simulink model "Long_Transmission_Line_Model"  (R2024b)
settings: Solver=VariableStepAuto  StartTime=0.0  StopTime=0.1  RelTol=1e-3
libraries: spsRMSLib x4, spsPower3phInstantaneousLib x2, spsThreePhaseVIMeasurementLib x2, spsDistributedParametersLineLib x1, spsThreePhaseSeriesRLCLoadLib x1, spsThreePhaseSourceLib x1, sps_lib x1
settings Model: Creator=vinaykumar7  LastModifiedBy=vinaykumar7

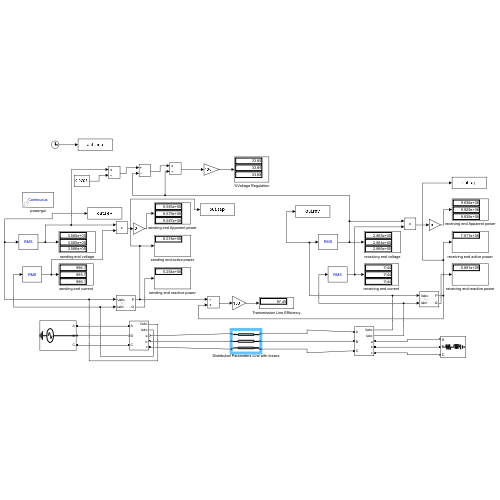
[thumbnail: Simulink's stored preview of the top-level diagram]
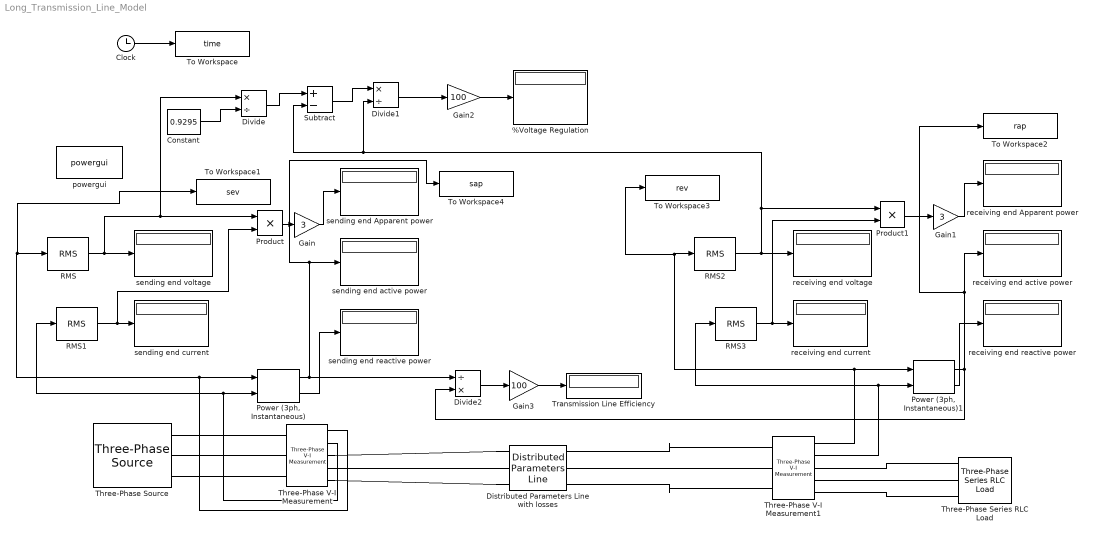
== system Long_Transmission_Line_Model ==
  %Voltage Regulation : Display
  Clock : Clock
  Constant : Constant  Value=0.9295
  Distributed Parameters Line with losses : spsDistributedParametersLineLib/Distributed Parameters Line  Phases=3  Length=300  Frequency=60  Resistance=[0.01 0.01]  Inductance="[0.97e-3  0.99e-3]"  Capacitance=[11.5e-9 11.5e-9]  x1=[5.82076609134674e-11 617530 617530;376.991118430775 376.991118430775 376.991118430775;1.18918707880175 0.426861843081656 -1.14393448371324]  x2=[5.82076609134674e-11 497009.835626798 497009.835626798;376.991118430775 376.991118430775 376.991118430775;-1.95240557478805 0.151474532002386 -1.41932179479251]  x3=[9.29377281793469e-13 1185.24504562472 1185.24504562472;376.991118430775 376.991118430775 376.991118430775;2.5297638183198 1.23233823295439 -0.338458093840513]  x4=[1.37600738157923e-12 3488.39051211722 3488.39051211722;376.991118430775 376.991118430775 376.991118430775;-0.216460570578523 -0.19563319043191 -1.76642951722681]  x5=0.00101224996912818  V1=[5.821e-11 6.175e+05 6.175e+05;377 377 377;1.189 0.4269 -1.144]  V2=[5.821e-11 4.97e+05 4.97e+05;377 377 377;-1.952 0.1515 -1.419]  I1=[9.294e-13 1185 1185;377 377 377;2.53 1.232 -0.3385]  I2=[1.376e-12 3488 3488;377 377 377;-0.2165 -0.1956 -1.766]  nHarmo=1  Measurements=None  Decoupling=off  VsMag0=0  VrMag0=0  VsAngle0=0  VrAngle0=0  IsMag0=0  IrMag0=0  IsAngle0=0  IrAngle0=0
      settings: LibrarySourceBlock=sps_lib/Power Grid Elements/Distributed Parameters Line
  Divide : Product  Inputs=*/
  Divide1 : Product  Inputs=*/
  Divide2 : Product  Inputs=/*
  Gain : Gain  Gain=3
  Gain1 : Gain  Gain=3
  Gain2 : Gain  Gain=100
  Gain3 : Gain  Gain=100
  "Power (3ph, Instantaneous)" : spsPower3phInstantaneousLib/Power (3ph, Instantaneous)
  "Power (3ph, Instantaneous)1" : spsPower3phInstantaneousLib/Power (3ph, Instantaneous)
  Product : Product
  Product1 : Product
  RMS{,1..3} (4 alike) : spsRMSLib/RMS  TrueRMS=on  Freq=60  RMSInit=0  Ts=0
  Subtract : Sum  Inputs=+-
  Three-Phase Series RLC Load : spsThreePhaseSeriesRLCLoadLib/Three-Phase Series RLC Load  LConnTagsString=A|B|C  Configuration=Y (grounded)  NominalVoltage=500e3  Vabc=[1e3 1e3 1e3]  Vabcp=[1e3 1e3 1e3]  NominalFrequency=60  UnbalancedPower=off  ActivePower=800e6  InductivePower=600e6  CapacitivePower=0  Pabc=[10e3 9e3 11e3]  QLabc=[100 90 110]  QCabc=[100 90 110]  Pabcp=[10e3 9e3 11e3]  QLabcp=[100 90 110]  QCabcp=[100 90 110]  Measurements=None  LoadType=constant Z
  Three-Phase V-I Measurement : spsThreePhaseVIMeasurementLib/Three-Phase V-I Measurement  VoltageMeasurement=phase-to-ground  SetLabelV=off  LabelV=Vabc  Vpu=off  VpuLL=off  CurrentMeasurement=yes  SetLabelI=off  LabelI=Iabc  Ipu=off  Pbase=100e6  Vbase=500e3  OutputType=Complex  PhasorSimulation=off  PSBequivalent=0
  Three-Phase V-I Measurement1 : spsThreePhaseVIMeasurementLib/Three-Phase V-I Measurement  VoltageMeasurement=phase-to-ground  SetLabelV=off  LabelV=Vabc  Vpu=off  VpuLL=off  CurrentMeasurement=yes  SetLabelI=off  LabelI=Iabc  Ipu=off  Pbase=100e6  Vbase=500e3  OutputType=Complex  PhasorSimulation=off  PSBequivalent=0
  Three-Phase Source : spsThreePhaseSourceLib/Three-Phase Source  InternalConnection=Yg  VoltagePhases=off  Voltage=617.53e3  PhaseAngle=16.1  Voltage_phases=[25e3 25e3 25e3]/sqrt(3)  PhaseAngles_phases=[0 -120 +120]  Frequency=60  NonIdealSource=off  SpecifyImpedance=off  Resistance=0.8929  Inductance=16.58e-3  ShortCircuitLevel=100e6  BaseVoltage=25e3  XRratio=7  BusType=swing  Pref=10e3  Qref=0  Prefabc=[10e3, 10e3, 10e3]  Qrefabc=[0, 0, 0]  Qmin=-inf  Qmax=inf
  To Workspace : ToWorkspace  VariableName=time  SampleTime=-1
      settings: Save2DSignal=2-D array (concatenate along first dimension)
  To Workspace1 : ToWorkspace  VariableName=sev  SampleTime=-1
      settings: Save2DSignal=2-D array (concatenate along first dimension)
  To Workspace2 : ToWorkspace  VariableName=rap  SampleTime=-1
      settings: Save2DSignal=2-D array (concatenate along first dimension)
  To Workspace3 : ToWorkspace  VariableName=rev  SampleTime=-1
      settings: Save2DSignal=2-D array (concatenate along first dimension)
  To Workspace4 : ToWorkspace  VariableName=sap  SampleTime=-1
      settings: Save2DSignal=2-D array (concatenate along first dimension)
  Transmission Line Efficiency : Display
  powergui : sps_lib/powergui  Priority=1  SimulationMode=Continuous  SampleTime=50e-6  frequency=60  Iterations=50  frequencyindice=60  Pbase=100e6  ErrMax=1e-4  UnitsV=kV  UnitsW=MW  buscounter=0  FunctionMessages=off  echomessages=off  EnableUseOfTLC=off  CurrentSourceSwitches=off  DisableSnubberDevices=off  DisableRonSwitches=off  DisableVfSwitches=off  DisplayEquations=off  AutomaticDiscreteSolvers=off  SolverType=Tustin/Backward Euler (TBE)  Interpol=off  ExternalGateDelay=off  methode=off  Ts=100  x0status=blocks  SPID=on  SwTol=0  HookPort=off  NonlinearTolerance=1e-4  nMaxIteration=100  ContinueOnMaxIteration=off  RestoreLinks=warning  ResistiveCurrentMeasurement=off  Frange=[0:2:500]  Ylog=off  Xlog=on  ShowGrid=off  save=off  variable=ZData  structure=0  ZoomFFT=off  StartTime=0.0  cycles=1  DisplayStyle=1  fundamental=60  FreqAxis=off  MaxFrequency=1000  frequencyindicesteady=1  RmsSteady=1  display=off
  receiving end Apparent power : Display
  receiving end active power : Display
  receiving end current : Display
  receiving end reactive power : Display
  receiving end voltage : Display
  sending end Apparent power : Display
  sending end active power : Display
  sending end current : Display
  sending end reactive power : Display
  sending end voltage : Display
  wires:
  Three-Phase V-I Measurement/1 -> "Power (3ph, Instantaneous)"/1, To Workspace1/1, RMS/1
  Three-Phase V-I Measurement/2 -> "Power (3ph, Instantaneous)"/2, RMS1/1
  RMS1/1 -> Product/2, sending end current/1
  "Power (3ph, Instantaneous)"/1 -> Divide2/1, sending end active power/1, To Workspace4/1
  "Power (3ph, Instantaneous)"/2 -> sending end reactive power/1
  Product/1 -> Gain/1
  Gain/1 -> sending end Apparent power/1
  Product1/1 -> Gain1/1
  Three-Phase V-I Measurement1/1 -> "Power (3ph, Instantaneous)1"/1, To Workspace3/1, RMS2/1
  Three-Phase V-I Measurement1/2 -> "Power (3ph, Instantaneous)1"/2, RMS3/1
  RMS3/1 -> Product1/2, receiving end current/1
  Gain1/1 -> receiving end Apparent power/1
  "Power (3ph, Instantaneous)1"/2 -> receiving end reactive power/1
  "Power (3ph, Instantaneous)1"/1 -> To Workspace2/1, receiving end active power/1, Divide2/2
  Constant/1 -> Divide/2
  Divide/1 -> Subtract/1
  Subtract/1 -> Divide1/1
  Divide1/1 -> Gain2/1
  Gain2/1 -> %Voltage Regulation/1
  Divide2/1 -> Gain3/1
  Gain3/1 -> Transmission Line Efficiency/1
  RMS/1 -> Divide/1, Product/1, sending end voltage/1
  RMS2/1 -> Divide1/2, Subtract/2, Product1/1, receiving end voltage/1
  Clock/1 -> To Workspace/1
  connections:
  Three-Phase Source/RConn1 -- Three-Phase V-I Measurement/LConn1
  Three-Phase Source/RConn2 -- Three-Phase V-I Measurement/LConn2
  Three-Phase Source/RConn3 -- Three-Phase V-I Measurement/LConn3
  Distributed Parameters Line with losses/LConn1 -- Three-Phase V-I Measurement/RConn1
  Distributed Parameters Line with losses/LConn2 -- Three-Phase V-I Measurement/RConn2
  Distributed Parameters Line with losses/LConn3 -- Three-Phase V-I Measurement/RConn3
  Three-Phase V-I Measurement1/LConn2 -- Distributed Parameters Line with losses/RConn2
  Distributed Parameters Line with losses/RConn1 -- Three-Phase V-I Measurement1/LConn1
  Distributed Parameters Line with losses/RConn3 -- Three-Phase V-I Measurement1/LConn3
  Three-Phase Series RLC Load/LConn2 -- Three-Phase V-I Measurement1/RConn2
  Three-Phase Series RLC Load/LConn1 -- Three-Phase V-I Measurement1/RConn1
  Three-Phase V-I Measurement1/RConn3 -- Three-Phase Series RLC Load/LConn3
